simulink model "ArduinoTest"  (R2019a)
settings: Solver=FixedStepAuto  StartTime=0.0  StopTime=inf  RelTol=1e-3  EnableMultiTasking=on
libraries: arduinolib x7
settings Model: SimulationMode=external  ExtModeTrigDuration=2  Creator=Safet  LastModifiedBy=Safet
settings OptimizationCC: EnhancedBackFolding=on  PassReuseOutputArgsAs=Individual arguments  MaxStackSize=64  OptimizeBlockOrder=speed  DifferentSizesBufferReuse=on  OptimizationCustomize=off
settings DebuggingCC: ParameterTunabilityLossMsg=error
settings HardwareCC: ProdBitPerInt=16  ProdBitPerPointer=16  ProdBitPerSizeT=16  ProdBitPerPtrDiffT=16  ProdLargestAtomicFloat=None  ProdWordSize=8  ProdHWDeviceType=Atmel->AVR
settings SFSimCC: MATLABDynamicMemAlloc=off
settings RTWCC: SystemTargetFile=ert.tlc  HardwareBoard=Arduino Uno  TLCOptions=-aInlineSetEventsForThisBaseRateFcn=TLC_FALSE -aSuppressMultiTaskScheduler=TLC_FALSE -aRateBasedStepFcn=1  TemplateMakefile=ert_default_tmf  GenerateReport=on  Toolchain=Arduino AVR  BuildConfiguration=Faster Runs  IncludeHyperlinkInReport=on  LaunchReport=on  GenerateTraceInfo=on  GenerateTraceReport=on  GenerateTraceReportSl=on  GenerateTraceReportSf=on  GenerateTraceReportEml=on
settings CodeAppCC: ForceParamTrailComments=on  IgnoreCustomStorageClasses=off  OperatorAnnotations=on  SimulinkDataObjDesc=on  SFDataObjDesc=on  InsertBlockDesc=on
settings ERTTargetCC: SupportContinuousTime=on  SupportVariableSizeSignals=on  ExtModeStaticAllocSize=250

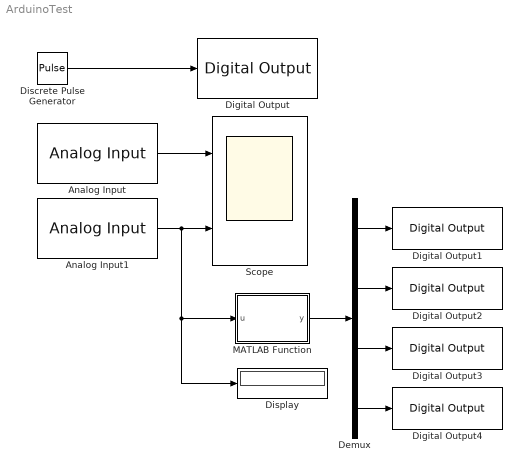
== system ArduinoTest ==
  Analog Input : arduinolib/Analog Input  pinNumber=0  ReadResultsOnly=off  ConversionTriggerSource=Software  ExternalTriggerType=uint32(0)  OutputDataType=uint16  EnableConversionCompleteNotify=off  EnableOuputStatus=off  SampleTime=0.01  blockPlatform=arduino
  Analog Input1 : arduinolib/Analog Input  pinNumber=2  ReadResultsOnly=off  ConversionTriggerSource=Software  ExternalTriggerType=uint32(0)  OutputDataType=uint16  EnableConversionCompleteNotify=off  EnableOuputStatus=off  SampleTime=0.01  blockPlatform=arduino
  Demux : Demux
  Digital Output : arduinolib/Digital Output  pinNumber=6  blockPlatform=arduino
  Digital Output1 : arduinolib/Digital Output  pinNumber=2  blockPlatform=arduino
  Digital Output2 : arduinolib/Digital Output  pinNumber=3  blockPlatform=arduino
  Digital Output3 : arduinolib/Digital Output  pinNumber=4  blockPlatform=arduino
  Digital Output4 : arduinolib/Digital Output  pinNumber=5  blockPlatform=arduino
  Discrete Pulse Generator : DiscretePulseGenerator  PulseType=Time based  Amplitude=0  Period=1  PulseWidth=50  VectorParams1D=off
  Display : Display
  MATLAB Function : MATLAB Function  TreatAsAtomicUnit=on
  Scope : Scope  NumInputPorts=2
  wires:
  Discrete Pulse Generator/1 -> Digital Output/1
  Analog Input/1 -> Scope/1
  Analog Input1/1 -> Display/1, MATLAB Function/1(u), Scope/2
  MATLAB Function/1(y) -> Demux/1
  Demux/4 -> Digital Output4/1
  Demux/3 -> Digital Output3/1
  Demux/2 -> Digital Output2/1
  Demux/1 -> Digital Output1/1

== matlab function ArduinoTest/MATLAB Function ==
  data: u input; y output
function y = fcn(u)    
    if u > 800
        y = [0 0 0 1];
    elseif u > 600
        y = [0 0 1 1];
    elseif u > 400
        y = [0 1 1 1];
    elseif u > 200
        y = [1 1 1 1];
    else
        y = [0 0 0 0];
    end
end
